simulink model "ControlSystemVoltChange"  (R2023a)
settings: Solver=VariableStepAuto  StartTime=0.0  StopTime=5.0  RelTol=1e-3
values from neighbouring files (symbols this model uses):
  ADC = (1/3.3)    (= 0.30303030303)    [Lab3_Student_Code_Motor02.m]
  denom = [J*L (J*R)+(B*L) (R*B)+K^2]    [Lab3_Student_Code_Motor02.m]
  DutyC = 1    [Lab3_Student_Code_Motor02.m]
  FV = 0.0022    [Lab3_Student_Code_Motor02.m]
  GR = (1/7.5)    (= 0.133333333333)    [Lab3_Student_Code_Motor02.m]
  Ki = (-wc)*(magGforward^-1)*sin(pi+wm-angleGforward)    [Lab3_Student_Code_Motor02.m]
  Kp = (magGforward^-1)*cos(pi+wm-angleGforward)    [Lab3_Student_Code_Motor02.m]
  num = K    (= 0.0621)    [Lab3_Student_Code_Motor02.m]
  RH = 16/(2*pi)    (= 2.54647908947)    [Lab3_Student_Code_Motor02.m]
  Ti = 1E3    (= 1000)    [Lab3_Student_Code_Motor02.m]
  Vbat = 7.2    [Lab3_Student_Code_Motor02.m]
settings Model: Creator=NG22  LastModifiedBy=NG22

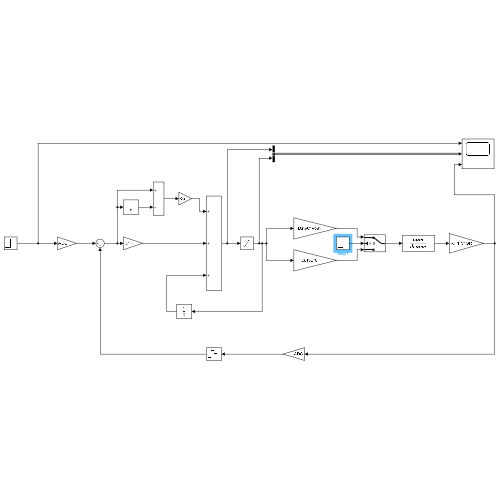
[thumbnail: Simulink's stored preview of the top-level diagram]
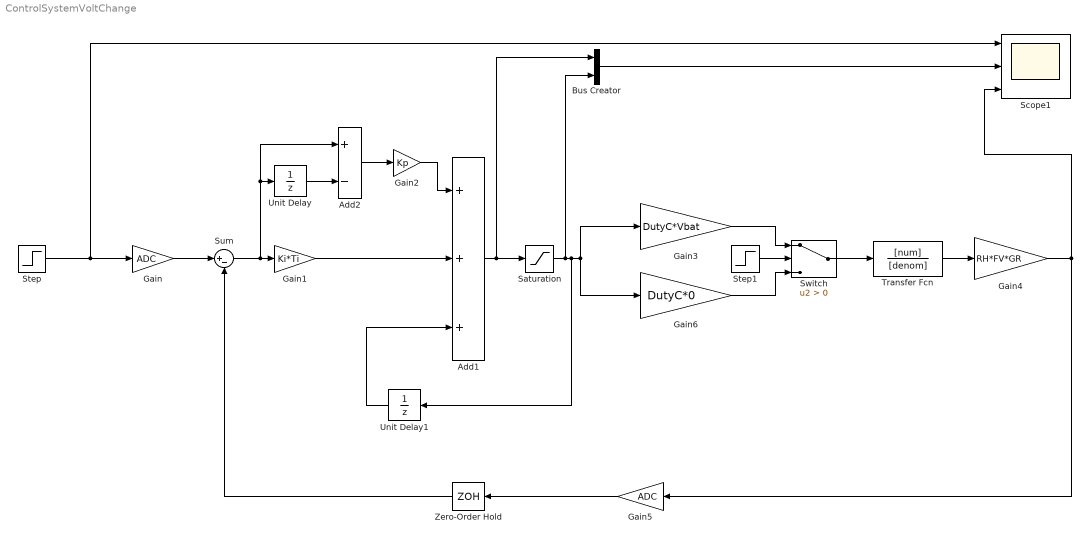
== system ControlSystemVoltChange ==
  Add1 : Sum  Inputs=+++
  Add2 : Sum  Inputs=+-
  Bus Creator : BusCreator  Inputs=2
  Gain : Gain  Gain=ADC
  Gain1 : Gain  Gain=Ki*Ti
  Gain2 : Gain  Gain=Kp
  Gain3 : Gain  Gain=DutyC*Vbat
  Gain4 : Gain  Gain=RH*FV*GR
  Gain5 : Gain  Gain=ADC
  Gain6 : Gain  Gain=DutyC*0
  Saturation : Saturate
  Scope1 : Scope  NumInputPorts=3
  Step : Step  SampleTime=0
  Step1 : Step  Time=3  SampleTime=0
  Sum : Sum  Inputs=|+-
  Switch : Switch  Criteria=u2 > Threshold  SaturateOnIntegerOverflow=off  InputSameDT=off
  Transfer Fcn : TransferFcn  Numerator=[num]  Denominator=[denom]
  Unit Delay : UnitDelay  SampleTime=-1  HasFrameUpgradeWarning=on
  Unit Delay1 : UnitDelay  SampleTime=-1  HasFrameUpgradeWarning=on
  Zero-Order Hold : ZeroOrderHold  SampleTime=-1
  wires:
  Step/1 -> Scope1/1, Gain/1
  Gain/1 -> Sum/1
  Sum/1 -> Gain1/1, Unit Delay/1, Add2/1
  Unit Delay/1 -> Add2/2
  Add2/1 -> Gain2/1
  Gain2/1 -> Add1/1
  Unit Delay1/1 -> Add1/3
  Saturation/1 -> Unit Delay1/1, Gain6/1, Gain3/1, Bus Creator/2
  Transfer Fcn/1 -> Gain4/1
  Add1/1 -> Bus Creator/1, Saturation/1
  Bus Creator/1 -> Scope1/2
  Gain4/1 -> Gain5/1, Scope1/3
  Gain5/1 -> Zero-Order Hold/1
  Zero-Order Hold/1 -> Sum/2
  Gain1/1 -> Add1/2
  Gain6/1 -> Switch/3
  Gain3/1 -> Switch/1
  Step1/1 -> Switch/2
  Switch/1 -> Transfer Fcn/1
